simulink model "adaptiveTest123"  (R2023a)
settings: Solver=FixedStepDiscrete  StartTime=0.0  StopTime=10.0  RelTol=1e-3
values from neighbouring files (symbols this model uses):
  a_coef = gain*reshape((1:M*K), M*K, 1).*ones(M*K,1)    [params.m]
  K = 1    [params.m]
  M = 1    [params.m]
libraries: commdigbbndam3 x1, commrandsrc3 x1, dspbuff3 x1
settings Model: DataTypeOverride=Off  Creator=dushe  LastModifiedBy=dushe
settings SolverCC: AlgebraicLoopSolver=TrustRegion
settings DataIOCC: LimitDataPoints=on  SaveOutput=off  SaveTime=off
settings OptimizationCC: BlockReduction=off  ConditionallyExecuteInputs=off  DefaultParameterBehavior=Inlined  LifeSpan=inf
settings DebuggingCC: AlgebraicLoopMsg=error  SingleTaskRateTransMsg=error  UnconnectedInputMsg=warning  UnconnectedOutputMsg=warning  UnconnectedLineMsg=warning  AllowSymbolicDim=off  StrictBusMsg=ErrorOnBusTreatedAsVector  SFUnexpectedBacktrackingDiag=warning  SFNoUnconditionalDefaultTransitionDiag=warning  SFExecutionAtInitializationDiag=none  ArithmeticOperatorsInVariantConditions=warning
settings HardwareCC: ProdBitPerPointer=32  ProdBitPerSizeT=32  ProdBitPerPtrDiffT=32  ProdLargestAtomicFloat=None  ProdIntDivRoundTo=Undefined  ProdEndianess=Unspecified  ProdWordSize=32  ProdHWDeviceType=ASIC/FPGA->ASIC/FPGA  ProdEqTarget=off
settings ModelReferenceCC: EnableRefExpFcnMdlSchedulingChecks=on
settings SFSimCC: SimUseLocalCustomCode=off  CustomCodeUndefinedFunction=UseInterfaceOnly
settings RTWCC: RTWUseLocalCustomCode=off
settings CodeAppCC: StateflowObjectComments=on
settings GRTTargetCC: TargetLangStandard=C89/C90 (ANSI)
settings ConfigComp: CovScope=ReferencedModels  CovMetricSettings=dw  CovSaveCumulativeToWorkspaceVar=on  CovSaveSingleToWorkspaceVar=on  CovExternalEMLEnable=off  CovSFcnEnable=off

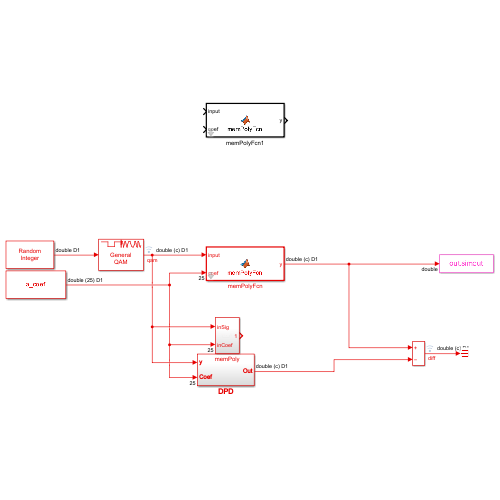
[thumbnail: Simulink's stored preview of the top-level diagram]
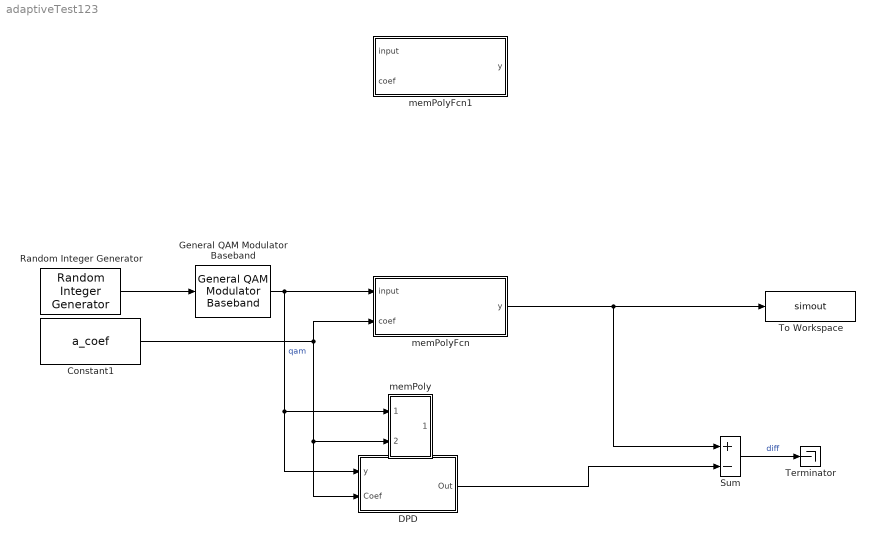
== system adaptiveTest123 ==
  Constant1 : Constant  Value=a_coef  SampleTime=-1
  DPD : Subsystem
  General QAM Modulator Baseband : commdigbbndam3/General QAM Modulator Baseband  SigCon=[exp(2*pi*1i*[0:3]/4 + 2*pi*1i/8)]  outDtype=double  outWordLen=16  outUDDataType=sfix(16)  outFracLenMode=Best precision  outFracLen=15  outDataTypeStr=double  outLastDataTypeStr=double
  Random Integer Generator : commrandsrc3/Random Integer Generator  SetSize=4  SeedSource=Auto  Seed=0  SampleTime=1  SamplesPerFrame=1  OutputDataType=double  SimulateUsing=Interpreted execution
  Sum : Sum  Inputs=+-
  Terminator : Terminator
  To Workspace : ToWorkspace  VariableName=simout  SaveFormat=Structure  SampleTime=-1
      settings: Save2DSignal=2-D array (concatenate along first dimension)
  memPoly : Subsystem
  memPolyFcn : MATLAB Function  TreatAsAtomicUnit=on  mask{M=M, K=K}
  memPolyFcn1 : MATLAB Function  TreatAsAtomicUnit=on  mask{M=M, K=K}
  wires:
  Random Integer Generator/1 -> General QAM Modulator Baseband/1
  Constant1/1 -> DPD/2(Coef), memPoly/2(inCoef), memPolyFcn/2(coef)
  General QAM Modulator Baseband/1 -> DPD/1(y), memPoly/1(inSig), memPolyFcn/1(input)  "qam"
  Sum/1 -> Terminator/1  "diff"
  DPD/1(Out) -> Sum/2
  memPolyFcn/1(y) -> To Workspace/1, Sum/1

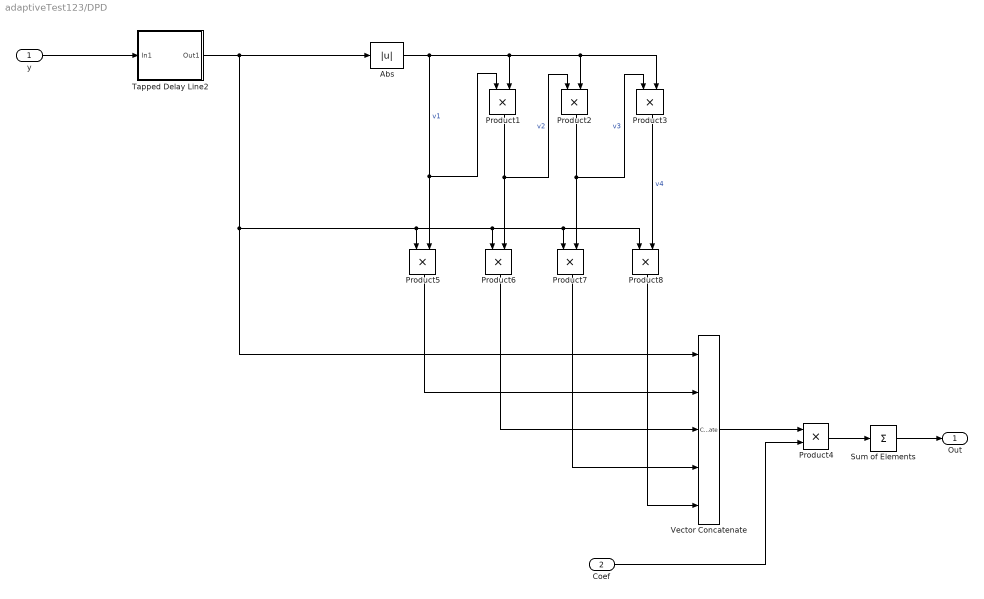
== system adaptiveTest123/DPD ==
  y : Inport
  Coef : Inport  Port=2
  Abs : Abs  SaturateOnIntegerOverflow=off
  Product{1..3,5..8} (7 alike) : Product  RndMeth=Zero
  Product4 : Product  OutDataTypeStr=double
  Sum of Elements : Sum  Inputs=+  OutDataTypeStr=double
  Tapped Delay Line2 : Subsystem
  Vector Concatenate : Concatenate  NumInputs=5
  Out : Outport
  wires:
  Sum of Elements/1 -> Out/1
  Coef/1 -> Product4/2
  Vector Concatenate/1 -> Product4/1
  Product4/1 -> Sum of Elements/1
  Abs/1 -> Product3/2, Product2/2, Product1/2, Product1/1, Product5/2  "v1"
  Product1/1 -> Product2/1, Product6/2  "v2"
  Product2/1 -> Product3/1, Product7/2  "v3"
  Product3/1 -> Product8/2  "v4"
  Product5/1 -> Vector Concatenate/2
  Product6/1 -> Vector Concatenate/3
  Product7/1 -> Vector Concatenate/4
  Product8/1 -> Vector Concatenate/5
  Tapped Delay Line2/1(Out1) -> Abs/1, Product8/1, Product7/1, Product6/1, Product5/1, Vector Concatenate/1
  y/1 -> Tapped Delay Line2/1(In1)

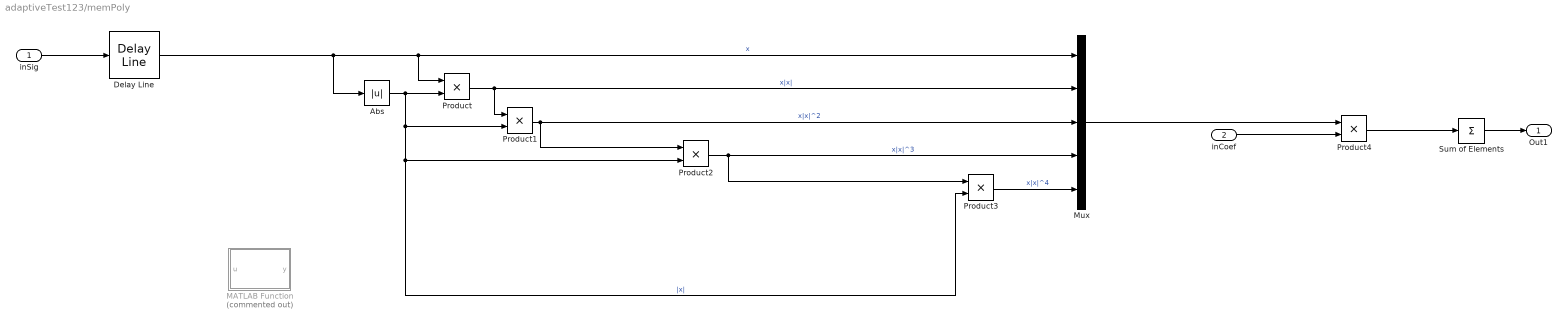
== system adaptiveTest123/memPoly ==
  inSig : Inport
  inCoef : Inport  Port=2
  Abs : Abs  SaturateOnIntegerOverflow=off
  Delay Line : dspbuff3/Delay Line  siz=5  ic=0  directfeed=on  enable_output=off  hold_output=off  OutputFrames=off
  MATLAB Function : MATLAB Function  Commented=on  TreatAsAtomicUnit=on
  Mux : Mux  Inputs=5
  Product{,1..4} (5 alike) : Product
  Sum of Elements : Sum  Inputs=+
  Out1 : Outport
  wires:
  Abs/1 -> Product3/2, Product2/2, Product1/2, Product/2  "|x|"
  Product3/1 -> Mux/5  "x|x|^4"
  Product1/1 -> Product2/1, Mux/3  "x|x|^2"
  Product4/1 -> Sum of Elements/1
  Product/1 -> Product1/1, Mux/2  "x|x|"
  Product2/1 -> Product3/1, Mux/4  "x|x|^3"
  Sum of Elements/1 -> Out1/1
  Mux/1 -> Product4/1
  inCoef/1 -> Product4/2
  Delay Line/1 -> Abs/1, Product/1, Mux/1  "x"
  inSig/1 -> Delay Line/1

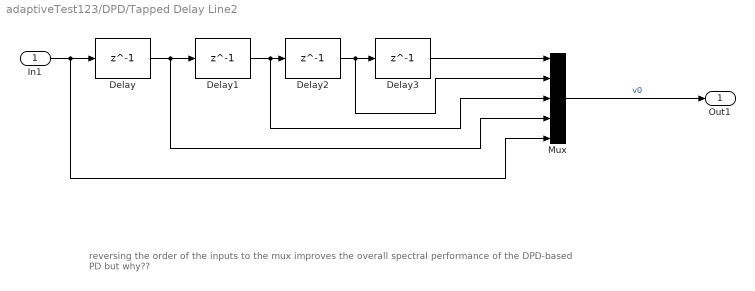
== system adaptiveTest123/DPD/Tapped Delay Line2 ==
  note: reversing the order of the inputs to the mux improves the overall spectral performance of the DPD-based PD but why??
  In1 : Inport
  Delay{,1..3} (4 alike) : Delay  DelayLength=1  InitialCondition=0  UseCircularBuffer=on
  Mux : Mux  Inputs=5
  Out1 : Outport
  wires:
  Delay3/1 -> Mux/1
  Mux/1 -> Out1/1  "v0"
  Delay2/1 -> Mux/2, Delay3/1
  Delay1/1 -> Mux/3, Delay2/1
  Delay/1 -> Mux/4, Delay1/1
  In1/1 -> Mux/5, Delay/1

== matlab function adaptiveTest123/memPolyFcn ==
  data: input input; y output; coef input; M parameter; K parameter
function y = memPolyFcn(input, coef, M, K)
persistent dataVector;
if isempty(dataVector)
    dataVector = zeros(M, 1, 'like', input);
end
%% shift delay register
dataVector(1:M-1) = dataVector(2:M);
dataVector(M) = input;

%% reshape coef
coef = reshape(coef, M, K);
%%
y = zeros(1, 1, 'like', input);
for k = 0:K-1
    for m = 0:M-1
        y = y + coef(1+m, 1+k)*dataVector(1+m)*abs(dataVector(1+m))^k;
    end
end

== matlab function adaptiveTest123/memPoly/MATLAB Function ==
  data: u input; y output
function y = fcn(u)
y = flip(u);

== matlab function adaptiveTest123/memPolyFcn1 ==
  data: input input; y output; coef input; M parameter; K parameter
function y = memPolyFcn(input, coef, M, K)
persistent dataVector;
if isempty(dataVector)
    dataVector = zeros(M, 1, 'like', input);
end
%% shift delay register
dataVector(1:M-1) = dataVector(2:M);
dataVector(M) = input;

%% reshape coef
coef = reshape(coef, M, K);
%%
y = zeros(1, 1, 'like', input);
for k = 0:K-1
    for m = 0:M-1
        y = y + coef(1+m, 1+k)*dataVector(1+m)*abs(dataVector(1+m))^k;
    end
end
